simulink model "zadatak2PID"  (R2018a)
settings: Solver=VariableStepAuto  StartTime=0.0  StopTime=50  RelTol=1e-3
values from neighbouring files (symbols this model uses):
  Kp = (1-exp(-T/Ts))/K0/(exp(T/T0) - 1)/(1 + N*(1 - exp(-T/Ts)))    [Parametri.m]
  T = 1    [Parametri.m]
undefined symbols (not defined in the file or in its folder): Td, Ti
settings Model: Creator=User  LastModifiedBy=User

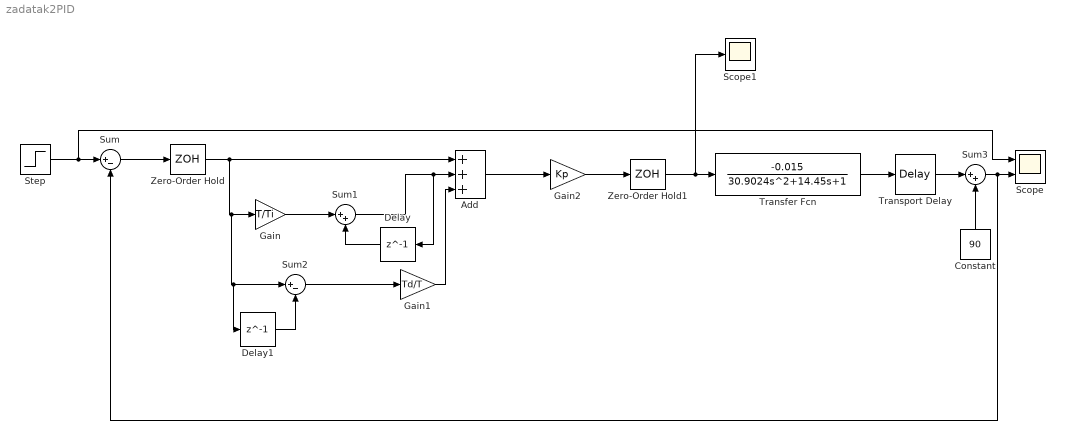
== system zadatak2PID ==
  Add : Sum  Inputs=+++
  Constant : Constant  Value=90
  Delay : Delay  DelayLength=1
  Delay1 : Delay  DelayLength=1
  Gain : Gain  Gain=T/Ti
  Gain1 : Gain  Gain=Td/T
  Gain2 : Gain  Gain=Kp
  Scope : Scope  NumInputPorts=2
  Scope1 : Scope
  Step : Step  Time=5  Before=90  After=80  SampleTime=0
  Sum : Sum  Inputs=|+-
  Sum1 : Sum  Inputs=|++
  Sum2 : Sum  Inputs=|+-
  Sum3 : Sum  Inputs=|++
  Transfer Fcn : TransferFcn  Numerator=[-0.015]  Denominator=[30.9024 14.45 1]
  Transport Delay : TransportDelay
  Zero-Order Hold : ZeroOrderHold
  Zero-Order Hold1 : ZeroOrderHold
  wires:
  Step/1 -> Scope/1, Sum/1
  Sum/1 -> Zero-Order Hold/1
  Zero-Order Hold/1 -> Delay1/1, Sum2/1, Gain/1, Add/1
  Gain/1 -> Sum1/1
  Sum1/1 -> Delay/1, Add/2
  Delay/1 -> Sum1/2
  Delay1/1 -> Sum2/2
  Sum2/1 -> Gain1/1
  Gain1/1 -> Add/3
  Add/1 -> Gain2/1
  Gain2/1 -> Zero-Order Hold1/1
  Zero-Order Hold1/1 -> Scope1/1, Transfer Fcn/1
  Transfer Fcn/1 -> Transport Delay/1
  Transport Delay/1 -> Sum3/1
  Constant/1 -> Sum3/2
  Sum3/1 -> Sum/2, Scope/2
